simulink model "modelsimulator"  (R2023b)
settings: Solver=VariableStepAuto  StartTime=0.0  StopTime=185  FixedStep=0.0002  RelTol=1e-3
values from neighbouring files (symbols this model uses):
  eta_init = [0 0 0 0 0 0]    [Linearization_validation.m]    (also in ROV_simulation_init.m = [radius 0 0 0 0 -pi/2])
  K_full = lqr(linsysROV_lqr,Q,R)    [ROV_simulation_init.m]
  K_reduced = lqr(linsysROV_lqr_reduced_disc,Q,R)    [ROV_simulation_init.m]
  omega = 0.0174532925*5    (= 0.0872664625)    [ROV_simulation_init.m]
  p = [-125.691529893755	-8.50647884753240	275.922008410927	13.4112646958028	-226.567986780204	-3.28875901062827	118.657519470084	6.62648580653865	14.9826070833980	0.00]    [ROV_simulation_init.m]
  PID_phi = [11.6676, 5.8503, -12.3688, 0.025226,34]    [ROV_simulation_init.m]
  PID_psi = [11.3054, 1.000, -3.8005, 0.087502,30]    [ROV_simulation_init.m]
  PID_theta = [10.2974, 5.9702, -15.653, 0.016423,19]    [ROV_simulation_init.m]
  PID_x = [500.411, 30.5093, -500.8638, 0.032394,110]    [ROV_simulation_init.m]
  PID_y = [500.7275, 20.1075, -500.8002, 0.019369,110]    [ROV_simulation_init.m]
  PID_z = [500.7655, 25.0859, -500.5557, 0.026709,158]    [ROV_simulation_init.m]
  radius = 5    [ROV_simulation_init.m]
  ROV = initializeModelMatrices(m,I,COG,l,w,h,Thrusters)    [CreateGramianROV.m]    (also in CreateROVLin.m = initializeModelMatrices(m, I, COB, dim, BlueROVHeavy); Eigenvalue_tracking.m = initializeModelMatrices(m, I, COB,dim,0); Linearization_validation.m = initializeModelMatrices(m, I, COB,dim,0); ROV_simulation_init.m = initializeModelMatrices(m, Inertia, COB, dim, BlueROVHeavy))
  T_inv = ROV.T'/(ROV.T*ROV.T')    [ROV_simulation_init.m]
  ThrusterVoltage = 14    [ROV_simulation_init.m]
  v_init = [3 0 0 0 0 0]    [Linearization_validation.m]    (also in ROV_simulation_init.m = [omega omega z_rate 0 0 omega])
  z_rate = 0.1    [ROV_simulation_init.m]
libraries: simulink x60
(part 3 of 3)

== matlab function modelsimulator/PID/Tau_body/InvNED ==
  data: Tau1 input; x_dot output; Tau2 input; Tau3 input; Tau4 input; Tau5 input; Tau6 input; x input; y input; z input; phi input; theta input; pzi input; y_dot output; z_dot output; phi_dot output; theta_dot output; pzi_dot output
function [x_dot,y_dot,z_dot,phi_dot,theta_dot,pzi_dot] = InvNED(Tau1,Tau2,Tau3,Tau4,Tau5,Tau6,x,y,z,phi,theta,pzi)
%#codegen

%    This function was generated by the Symbolic Math Toolbox version 23.2.
%    07-Jun-2024 11:07:48

% Tau1 = complex(Tau1);  % if required to enforce complex operations
% Tau2 = complex(Tau2);  % if required to enforce complex operations
% Tau3 = complex(Tau3);  % if required to enforce complex operations
% Tau4 = complex(Tau4);  % if required to enforce complex operations
% Tau5 = complex(Tau5);  % if required to enforce complex operations
% Tau6 = complex(Tau6);  % if required to enforce complex operations
% x = complex(x);  % if required to enforce complex operations
% y = complex(y);  % if required to enforce complex operations
% z = complex(z);  % if required to enforce complex operations
% phi = complex(phi);  % if required to enforce complex operations
% theta = complex(theta);  % if required to enforce complex operations
% pzi = complex(pzi);  % if required to enforce complex operations
t2 = cos(phi);
t3 = cos(pzi);
t4 = cos(theta);
t5 = sin(phi);
t6 = sin(pzi);
t7 = sin(theta);
t8 = t2.^2;
t9 = t3.^2;
t10 = t4.^2;
t11 = t5.^2;
t12 = t6.^2;
t13 = t7.^2;
t14 = t8.*t10;
t15 = t8+t11;
t16 = t9+t12;
t17 = t8.*t13;
t18 = t10.*t11;
t19 = t11.*t13;
t20 = 1.0./t15;
t21 = 1.0./t16;
x_dot = (t21.*(Tau1.*t3.*t4+Tau2.*t4.*t6-Tau3.*t7.*t9-Tau3.*t7.*t12))./(t10+t13);
if nargout > 1
    t22 = t14+t17+t18+t19;
    t23 = 1.0./t22;
    y_dot = t21.*t23.*(Tau1.*t3.*t5.*t7+Tau2.*t2.*t3.*t10-Tau1.*t2.*t6.*t10+Tau2.*t2.*t3.*t13+Tau2.*t5.*t6.*t7+Tau3.*t4.*t5.*t9-Tau1.*t2.*t6.*t13+Tau3.*t4.*t5.*t12);
end
if nargout > 2
    z_dot = t21.*t23.*(Tau1.*t2.*t3.*t7+Tau2.*t2.*t6.*t7+Tau3.*t2.*t4.*t9-Tau2.*t3.*t5.*t10+Tau3.*t2.*t4.*t12+Tau1.*t5.*t6.*t10-Tau2.*t3.*t5.*t13+Tau1.*t5.*t6.*t13);
end
if nargout > 3
    phi_dot = Tau4-Tau6.*t4.*tan(theta);
end
if nargout > 4
    theta_dot = t20.*(Tau5.*t2+Tau6.*t4.*t5);
end
if nargout > 5
    pzi_dot = -t20.*(Tau5.*t5-Tau6.*t2.*t4);
end
end

== matlab function modelsimulator/LQR_full/Tau_body/InvNED ==
  data: Tau1 input; x_dot output; Tau2 input; Tau3 input; Tau4 input; Tau5 input; Tau6 input; x input; y input; z input; phi input; theta input; pzi input; y_dot output; z_dot output; phi_dot output; theta_dot output; pzi_dot output
function [x_dot,y_dot,z_dot,phi_dot,theta_dot,pzi_dot] = InvNED(Tau1,Tau2,Tau3,Tau4,Tau5,Tau6,x,y,z,phi,theta,pzi)
%#codegen

%    This function was generated by the Symbolic Math Toolbox version 23.2.
%    21-May-2024 16:03:04

% Tau1 = complex(Tau1);  % if required to enforce complex operations
% Tau2 = complex(Tau2);  % if required to enforce complex operations
% Tau3 = complex(Tau3);  % if required to enforce complex operations
% Tau4 = complex(Tau4);  % if required to enforce complex operations
% Tau5 = complex(Tau5);  % if required to enforce complex operations
% Tau6 = complex(Tau6);  % if required to enforce complex operations
% x = complex(x);  % if required to enforce complex operations
% y = complex(y);  % if required to enforce complex operations
% z = complex(z);  % if required to enforce complex operations
% phi = complex(phi);  % if required to enforce complex operations
% theta = complex(theta);  % if required to enforce complex operations
% pzi = complex(pzi);  % if required to enforce complex operations
t2 = cos(phi);
t3 = cos(pzi);
t4 = cos(theta);
t5 = sin(phi);
t6 = sin(pzi);
t7 = sin(theta);
t8 = t2.^2;
t9 = t3.^2;
t10 = t4.^2;
t11 = t5.^2;
t12 = t6.^2;
t13 = t7.^2;
t14 = t8.*t10;
t15 = t8+t11;
t16 = t9+t12;
t17 = t8.*t13;
t18 = t10.*t11;
t19 = t11.*t13;
t20 = 1.0./t15;
t21 = 1.0./t16;
x_dot = (t21.*(Tau1.*t3.*t4+Tau2.*t4.*t6-Tau3.*t7.*t9-Tau3.*t7.*t12))./(t10+t13);
if nargout > 1
    t22 = t14+t17+t18+t19;
    t23 = 1.0./t22;
    y_dot = t21.*t23.*(Tau1.*t3.*t5.*t7+Tau2.*t2.*t3.*t10-Tau1.*t2.*t6.*t10+Tau2.*t2.*t3.*t13+Tau2.*t5.*t6.*t7+Tau3.*t4.*t5.*t9-Tau1.*t2.*t6.*t13+Tau3.*t4.*t5.*t12);
end
if nargout > 2
    z_dot = t21.*t23.*(Tau1.*t2.*t3.*t7+Tau2.*t2.*t6.*t7+Tau3.*t2.*t4.*t9-Tau2.*t3.*t5.*t10+Tau3.*t2.*t4.*t12+Tau1.*t5.*t6.*t10-Tau2.*t3.*t5.*t13+Tau1.*t5.*t6.*t13);
end
if nargout > 3
    phi_dot = Tau4-Tau6.*t4.*tan(theta);
end
if nargout > 4
    theta_dot = t20.*(Tau5.*t2+Tau6.*t4.*t5);
end
if nargout > 5
    pzi_dot = -t20.*(Tau5.*t5-Tau6.*t2.*t4);
end
end

== matlab function modelsimulator/SMC/SMC_internal/SMC ==
  data: x input; Tau_1 output; y input; z input; phi input; theta input; pzi input; x_d input; y_d input; z_d input; phi_d input; theta_d input; pzi_d input; ref1 input; ref2 input; ref3 input; ref4 input; ref5 input; ref6 input; ref_d1 input; ref_d2 input; ref_d3 input; ref_d4 input; ref_d5 input; ref_d6 input; ref_dd1 input; ref_dd2 input; ref_dd3 input; ref_dd4 input; ref_dd5 input; ref_dd6 input; Tau_2 output; Tau_3 output; Tau_4 output; Tau_5 output; Tau_6 output; e_int1 input; e_int2 input; e_int3 input; e_int4 input; e_int5 input; e_int6 input; S_1 output; S_2 output; S_3 output; S_4 output; S_5 output; S_6 output
function [Tau_1,Tau_2,Tau_3,Tau_4,Tau_5,Tau_6,S_1,S_2,S_3,S_4,S_5,S_6] = SMC(x,y,z,phi,theta,pzi,x_d,y_d,z_d,phi_d,theta_d,pzi_d,ref1,ref2,ref3,ref4,ref5,ref6,ref_d1,ref_d2,ref_d3,ref_d4,ref_d5,ref_d6,ref_dd1,ref_dd2,ref_dd3,ref_dd4,ref_dd5,ref_dd6,e_int1,e_int2,e_int3,e_int4,e_int5,e_int6)
%#codegen

%    This function was generated by the Symbolic Math Toolbox version 23.2.
%    07-Jun-2024 11:09:30

% x = complex(x);  % if required to enforce complex operations
% y = complex(y);  % if required to enforce complex operations
% z = complex(z);  % if required to enforce complex operations
% phi = complex(phi);  % if required to enforce complex operations
% theta = complex(theta);  % if required to enforce complex operations
% pzi = complex(pzi);  % if required to enforce complex operations
% x_d = complex(x_d);  % if required to enforce complex operations
% y_d = complex(y_d);  % if required to enforce complex operations
% z_d = complex(z_d);  % if required to enforce complex operations
% phi_d = complex(phi_d);  % if required to enforce complex operations
% theta_d = complex(theta_d);  % if required to enforce complex operations
% pzi_d = complex(pzi_d);  % if required to enforce complex operations
% ref1 = complex(ref1);  % if required to enforce complex operations
% ref2 = complex(ref2);  % if required to enforce complex operations
% ref3 = complex(ref3);  % if required to enforce complex operations
% ref4 = complex(ref4);  % if required to enforce complex operations
% ref5 = complex(ref5);  % if required to enforce complex operations
% ref6 = complex(ref6);  % if required to enforce complex operations
% ref_d1 = complex(ref_d1);  % if required to enforce complex operations
% ref_d2 = complex(ref_d2);  % if required to enforce complex operations
% ref_d3 = complex(ref_d3);  % if required to enforce complex operations
% ref_d4 = complex(ref_d4);  % if required to enforce complex operations
% ref_d5 = complex(ref_d5);  % if required to enforce complex operations
% ref_d6 = complex(ref_d6);  % if required to enforce complex operations
% ref_dd1 = complex(ref_dd1);  % if required to enforce complex operations
% ref_dd2 = complex(ref_dd2);  % if required to enforce complex operations
% ref_dd3 = complex(ref_dd3);  % if required to enforce complex operations
% ref_dd4 = complex(ref_dd4);  % if required to enforce complex operations
% ref_dd5 = complex(ref_dd5);  % if required to enforce complex operations
% ref_dd6 = complex(ref_dd6);  % if required to enforce complex operations
% e_int1 = complex(e_int1);  % if required to enforce complex operations
% e_int2 = complex(e_int2);  % if required to enforce complex operations
% e_int3 = complex(e_int3);  % if required to enforce complex operations
% e_int4 = complex(e_int4);  % if required to enforce complex operations
% e_int5 = complex(e_int5);  % if required to enforce complex operations
% e_int6 = complex(e_int6);  % if required to enforce complex operations
t2 = abs(phi_d);
t3 = abs(pzi_d);
t4 = cos(phi);
t5 = cos(pzi);
t6 = abs(theta_d);
t7 = cos(theta);
t8 = abs(x_d);
t9 = abs(y_d);
t10 = abs(z_d);
t11 = sin(phi);
t12 = sin(pzi);
t13 = sin(theta);
t14 = tan(theta);
t15 = ref1.*2.0;
t16 = ref2.*2.0;
t17 = ref3.*2.0;
t18 = x.*2.0;
t19 = y.*2.0;
t20 = z.*2.0;
t35 = -ref_d1;
t36 = -ref_d2;
t37 = -ref_d3;
t38 = -ref_d4;
t39 = -ref_d5;
t40 = -ref_d6;
t41 = e_int6./2.0;
t42 = ref5.*(7.0./2.0);
t43 = theta.*(7.0./2.0);
t44 = e_int1.*(3.0./2.0e+1);
t45 = e_int2.*(3.0./2.0e+1);
t46 = e_int3.*(3.0./2.0e+1);
t48 = e_int4.*(9.0./1.0e+1);
t49 = e_int5.*(2.1e+1./2.0e+1);
t50 = phi.*(2.7e+1./1.0e+1);
t51 = pzi.*(1.3e+1./1.0e+1);
t52 = ref6.*(1.3e+1./1.0e+1);
t53 = ref4.*(2.7e+1./1.0e+1);
t21 = t4.^2;
t22 = t5.^2;
t23 = t5.^3;
t24 = t7.^2;
t25 = t7.^3;
t26 = t11.^2;
t27 = t11.^3;
t28 = t12.^2;
t29 = t12.^3;
t30 = t13.^2;
t31 = t13.^3;
t32 = -t15;
t33 = -t16;
t34 = -t17;
t47 = -t42;
t54 = -t52;
t55 = -t53;
t56 = t21+t26;
t58 = t21.*t22.*t30;
t59 = t21.*t24.*t28;
t60 = t22.*t24.*t26;
t61 = t4.*t5.*t11.*t12.*t31;
t62 = t5.*t7.*t11.*t12.*t31;
t63 = t5.*t11.*t12.*t13.*t25;
t64 = t22.*t26.*t30;
t65 = t24.*t26.*t28;
t66 = t26.*t28.*t30;
t67 = t4.*t7.*t28.*t30;
t68 = t21.*t22.*t24;
t71 = t4.*t5.*t11.*t12.*t13.*t24;
t72 = t18+t32+t35+t44+x_d;
t73 = t19+t33+t36+t45+y_d;
t74 = t20+t34+t37+t46+z_d;
t75 = t39+t43+t47+t49+theta_d;
t76 = pzi_d+t40+t41+t51+t54;
t77 = phi_d+t38+t48+t50+t55;
t57 = 1.0./t56;
t69 = -t62;
t70 = -t63;
t78 = t58+t59+t60+t61+t64+t65+t66+t67+t68+t69+t70+t71;
t79 = 1.0./t78;
et1 = t58.*x_d.*4.50486366e+9+t60.*x_d.*3.031307621e+9+t61.*x_d.*4.50486366e+9-t63.*x_d.*3.031307621e+9+t65.*x_d.*4.50486366e+9+t66.*x_d.*4.50486366e+9+t68.*x_d.*3.031307621e+9+t71.*x_d.*7.536171281e+9+t8.*t60.*x_d.*3.119812953e+10+t9.*t59.*x_d.*4.62422226e+10+t10.*t58.*x_d.*2.59370938e+10-t8.*t63.*x_d.*3.119812953e+10-t9.*t62.*x_d.*4.62422226e+10+t10.*t61.*x_d.*2.59370938e+10;
et2 = t9.*t64.*x_d.*4.62422226e+10+t10.*t65.*x_d.*2.59370938e+10+t8.*t68.*x_d.*3.119812953e+10+t9.*t67.*x_d.*4.62422226e+10+t10.*t66.*x_d.*2.59370938e+10+t8.*t71.*x_d.*3.119812953e+10-t9.*t71.*x_d.*4.62422226e+10+t10.*t71.*x_d.*2.59370938e+10+t4.*t11.*t13.*t28.*y_d.*4.50486366e+9+t5.*t12.*t21.*t24.*y_d.*3.031307621e+9-t5.*t12.*t24.*t26.*y_d.*1.473556039e+9-t4.*t11.*t22.*t31.*y_d.*4.50486366e+9;
et3 = t5.*t12.*t21.*t30.*y_d.*4.50486366e+9-t5.*t12.*t26.*t30.*y_d.*4.50486366e+9+t4.*t7.*t11.*t29.*z_d.*4.50486366e+9+t7.*t13.*t21.*t23.*z_d.*1.473556039e+9-t7.*t13.*t23.*t26.*z_d.*3.031307621e+9+t4.*t5.*t11.*t12.*t13.*x_d.*4.50486366e+9-t4.*t9.*t11.*t13.*t28.*y_d.*4.62422226e+10+t4.*t10.*t11.*t13.*t28.*y_d.*2.59370938e+10+t5.*t8.*t12.*t21.*t24.*y_d.*3.119812953e+10-t5.*t9.*t12.*t21.*t24.*y_d.*4.62422226e+10-t4.*t11.*t13.*t22.*t24.*y_d.*4.50486366e+9;
et4 = t5.*t8.*t12.*t24.*t26.*y_d.*3.119812953e+10+t4.*t9.*t11.*t22.*t31.*y_d.*4.62422226e+10-t5.*t9.*t12.*t21.*t30.*y_d.*4.62422226e+10-t5.*t10.*t12.*t24.*t26.*y_d.*2.59370938e+10-t4.*t10.*t11.*t22.*t31.*y_d.*2.59370938e+10+t5.*t10.*t12.*t21.*t30.*y_d.*2.59370938e+10+t5.*t9.*t12.*t26.*t30.*y_d.*4.62422226e+10-t5.*t10.*t12.*t26.*t30.*y_d.*2.59370938e+10+t4.*t7.*t11.*t12.*t22.*z_d.*4.50486366e+9-t4.*t7.*t9.*t11.*t29.*z_d.*4.62422226e+10;
et5 = t4.*t7.*t10.*t11.*t29.*z_d.*2.59370938e+10-t7.*t8.*t13.*t21.*t23.*z_d.*3.119812953e+10-t4.*t5.*t13.*t24.*t28.*z_d.*3.031307621e+9+t5.*t7.*t13.*t21.*t28.*z_d.*4.50486366e+9+t7.*t10.*t13.*t21.*t23.*z_d.*2.59370938e+10-t7.*t8.*t13.*t23.*t26.*z_d.*3.119812953e+10+t7.*t9.*t13.*t23.*t26.*z_d.*4.62422226e+10-t5.*t7.*t13.*t26.*t28.*z_d.*3.031307621e+9+t11.*t12.*t22.*t24.*t30.*z_d.*3.031307621e+9-t4.*t5.*t9.*t11.*t12.*t13.*x_d.*4.62422226e+10;
et6 = t4.*t5.*t10.*t11.*t12.*t13.*x_d.*2.59370938e+10+t4.*t9.*t11.*t13.*t22.*t24.*y_d.*4.62422226e+10-t4.*t10.*t11.*t13.*t22.*t24.*y_d.*2.59370938e+10-t4.*t7.*t9.*t11.*t12.*t22.*z_d.*4.62422226e+10+t4.*t7.*t10.*t11.*t12.*t22.*z_d.*2.59370938e+10-t4.*t5.*t8.*t13.*t24.*t28.*z_d.*3.119812953e+10+t4.*t5.*t9.*t13.*t24.*t28.*z_d.*4.62422226e+10-t5.*t7.*t9.*t13.*t21.*t28.*z_d.*4.62422226e+10+t5.*t7.*t10.*t13.*t21.*t28.*z_d.*2.59370938e+10-t4.*t7.*t11.*t12.*t22.*t30.*z_d.*3.031307621e+9;
et7 = t5.*t7.*t8.*t13.*t26.*t28.*z_d.*-3.119812953e+10+t5.*t7.*t9.*t13.*t26.*t28.*z_d.*4.62422226e+10+t8.*t11.*t12.*t22.*t24.*t30.*z_d.*3.119812953e+10-t9.*t11.*t12.*t22.*t24.*t30.*z_d.*4.62422226e+10-t4.*t7.*t8.*t11.*t12.*t22.*t30.*z_d.*3.119812953e+10+t4.*t7.*t9.*t11.*t12.*t22.*t30.*z_d.*4.62422226e+10;
Tau_1 = -(t72.*(abs(ref1.*(-3.0./2.0e+1)-ref_d1.*2.0+ref_dd1+x.*(3.0./2.0e+1)+x_d.*2.0+t79.*(et1+et2+et3+et4+et5+et6+et7).*2.275680623214713e-10).*(9.93e+2./5.0e+1)+9.93e+2./2.5e+1))./(abs(t72)+1.0./1.0e+1);
if nargout > 1
    et8 = t59.*y_d.*3.031307621e+9+t60.*y_d.*4.50486366e+9-t62.*y_d.*4.50486366e+9-t63.*y_d.*4.50486366e+9+t64.*y_d.*4.50486366e+9+t65.*y_d.*3.031307621e+9+t67.*y_d.*4.50486366e+9+t8.*t59.*y_d.*3.119812953e+10+t9.*t58.*y_d.*4.62422226e+10+t9.*t61.*y_d.*4.62422226e+10+t10.*t60.*y_d.*2.59370938e+10-t10.*t62.*y_d.*2.59370938e+10+t8.*t65.*y_d.*3.119812953e+10-t10.*t63.*y_d.*2.59370938e+10;
    et9 = t10.*t64.*y_d.*2.59370938e+10+t9.*t66.*y_d.*4.62422226e+10+t9.*t68.*y_d.*4.62422226e+10+t10.*t67.*y_d.*2.59370938e+10+t9.*t71.*y_d.*4.62422226e+10-t5.*t11.*t67.*z_d.*3.031307621e+9-t4.*t11.*t13.*t22.*x_d.*4.50486366e+9+t5.*t12.*t21.*t24.*x_d.*3.031307621e+9-t5.*t12.*t24.*t26.*x_d.*1.473556039e+9-t5.*t12.*t26.*t30.*x_d.*4.50486366e+9+t7.*t11.*t28.*t31.*x_d.*4.50486366e+9+t11.*t13.*t25.*t28.*x_d.*1.473556039e+9;
    et10 = t4.*t7.*t11.*t23.*z_d.*-4.50486366e+9+t4.*t13.*t24.*t29.*z_d.*1.473556039e+9-t7.*t13.*t26.*t29.*z_d.*3.031307621e+9-t5.*t8.*t11.*t67.*z_d.*3.119812953e+10+t5.*t9.*t11.*t67.*z_d.*4.62422226e+10+t4.*t5.*t7.*t12.*t30.*x_d.*4.50486366e+9+t4.*t9.*t11.*t13.*t22.*x_d.*4.62422226e+10-t4.*t10.*t11.*t13.*t22.*x_d.*2.59370938e+10+t5.*t8.*t12.*t21.*t24.*x_d.*3.119812953e+10-t5.*t9.*t12.*t21.*t24.*x_d.*4.62422226e+10+t5.*t8.*t12.*t24.*t26.*x_d.*3.119812953e+10;
    et11 = t5.*t10.*t12.*t24.*t26.*x_d.*-2.59370938e+10+t4.*t11.*t13.*t24.*t28.*x_d.*3.031307621e+9+t5.*t9.*t12.*t26.*t30.*x_d.*4.62422226e+10-t5.*t10.*t12.*t26.*t30.*x_d.*2.59370938e+10-t8.*t11.*t13.*t25.*t28.*x_d.*3.119812953e+10-t7.*t9.*t11.*t28.*t31.*x_d.*4.62422226e+10+t7.*t10.*t11.*t28.*t31.*x_d.*2.59370938e+10+t10.*t11.*t13.*t25.*t28.*x_d.*2.59370938e+10-t4.*t5.*t11.*t12.*t13.*y_d.*4.50486366e+9+t4.*t7.*t9.*t11.*t23.*z_d.*4.62422226e+10;
    et12 = t4.*t5.*t7.*t11.*t28.*z_d.*-4.50486366e+9-t4.*t7.*t10.*t11.*t23.*z_d.*2.59370938e+10+t4.*t12.*t13.*t22.*t24.*z_d.*4.50486366e+9-t7.*t12.*t13.*t21.*t22.*z_d.*3.031307621e+9-t4.*t8.*t13.*t24.*t29.*z_d.*3.119812953e+10+t4.*t10.*t13.*t24.*t29.*z_d.*2.59370938e+10-t7.*t12.*t13.*t22.*t26.*z_d.*3.031307621e+9-t7.*t8.*t13.*t26.*t29.*z_d.*3.119812953e+10+t7.*t9.*t13.*t26.*t29.*z_d.*4.62422226e+10+t5.*t11.*t24.*t28.*t30.*z_d.*3.031307621e+9;
    et13 = t4.*t5.*t7.*t9.*t12.*t30.*x_d.*-4.62422226e+10+t4.*t5.*t7.*t10.*t12.*t30.*x_d.*2.59370938e+10+t4.*t8.*t11.*t13.*t24.*t28.*x_d.*3.119812953e+10-t4.*t9.*t11.*t13.*t24.*t28.*x_d.*4.62422226e+10+t4.*t5.*t9.*t11.*t12.*t13.*y_d.*4.62422226e+10-t4.*t5.*t10.*t11.*t12.*t13.*y_d.*2.59370938e+10+t4.*t5.*t7.*t9.*t11.*t28.*z_d.*4.62422226e+10-t4.*t5.*t7.*t10.*t11.*t28.*z_d.*2.59370938e+10-t7.*t8.*t12.*t13.*t21.*t22.*z_d.*3.119812953e+10-t4.*t9.*t12.*t13.*t22.*t24.*z_d.*4.62422226e+10;
    et14 = t7.*t9.*t12.*t13.*t21.*t22.*z_d.*4.62422226e+10+t4.*t10.*t12.*t13.*t22.*t24.*z_d.*2.59370938e+10-t7.*t8.*t12.*t13.*t22.*t26.*z_d.*3.119812953e+10+t7.*t9.*t12.*t13.*t22.*t26.*z_d.*4.62422226e+10+t5.*t8.*t11.*t24.*t28.*t30.*z_d.*3.119812953e+10-t5.*t9.*t11.*t24.*t28.*t30.*z_d.*4.62422226e+10;
    Tau_2 = -(t73.*(abs(ref2.*(-3.0./2.0e+1)-ref_d2.*2.0+ref_dd2+y.*(3.0./2.0e+1)+y_d.*2.0+t79.*(et8+et9+et10+et11+et12+et13+et14).*2.275680623214713e-10).*2.0621e+1+4.124e+1))./(abs(t73)+1.0./1.0e+1);
end
if nargout > 2
    et15 = t58.*z_d.*3.031307621e+9+t59.*z_d.*4.50486366e+9+t61.*z_d.*3.031307621e+9-t62.*z_d.*3.031307621e+9+t64.*z_d.*3.031307621e+9+t66.*z_d.*3.031307621e+9+t67.*z_d.*3.031307621e+9+t68.*z_d.*4.50486366e+9+t8.*t58.*z_d.*3.119812953e+10+t8.*t61.*z_d.*3.119812953e+10+t9.*t60.*z_d.*4.62422226e+10+t10.*t59.*z_d.*2.59370938e+10-t8.*t62.*z_d.*3.119812953e+10+t8.*t64.*z_d.*3.119812953e+10;
    et16 = t9.*t63.*z_d.*-4.62422226e+10+t8.*t66.*z_d.*3.119812953e+10+t9.*t65.*z_d.*4.62422226e+10+t8.*t67.*z_d.*3.119812953e+10+t10.*t68.*z_d.*2.59370938e+10+t9.*t71.*z_d.*4.62422226e+10+t5.*t7.*t13.*t21.*x_d.*1.473556039e+9-t5.*t7.*t13.*t26.*x_d.*3.031307621e+9+t4.*t11.*t12.*t25.*x_d.*4.50486366e+9+t11.*t12.*t24.*t30.*x_d.*3.031307621e+9-t4.*t5.*t11.*t25.*y_d.*4.50486366e+9+t7.*t12.*t13.*t21.*y_d.*1.473556039e+9;
    et17 = t7.*t12.*t13.*t26.*y_d.*-3.031307621e+9-t5.*t7.*t8.*t13.*t21.*x_d.*3.119812953e+10+t5.*t7.*t10.*t13.*t21.*x_d.*2.59370938e+10-t5.*t7.*t8.*t13.*t26.*x_d.*3.119812953e+10+t5.*t7.*t9.*t13.*t26.*x_d.*4.62422226e+10-t4.*t9.*t11.*t12.*t25.*x_d.*4.62422226e+10+t4.*t10.*t11.*t12.*t25.*x_d.*2.59370938e+10+t4.*t7.*t11.*t12.*t30.*x_d.*1.473556039e+9+t8.*t11.*t12.*t24.*t30.*x_d.*3.119812953e+10-t9.*t11.*t12.*t24.*t30.*x_d.*4.62422226e+10+t4.*t5.*t9.*t11.*t25.*y_d.*4.62422226e+10;
    et18 = t4.*t5.*t10.*t11.*t25.*y_d.*-2.59370938e+10-t4.*t5.*t7.*t11.*t30.*y_d.*4.50486366e+9-t7.*t8.*t12.*t13.*t21.*y_d.*3.119812953e+10+t7.*t10.*t12.*t13.*t21.*y_d.*2.59370938e+10-t7.*t8.*t12.*t13.*t26.*y_d.*3.119812953e+10+t7.*t9.*t12.*t13.*t26.*y_d.*4.62422226e+10-t4.*t7.*t8.*t11.*t12.*t30.*x_d.*3.119812953e+10+t4.*t7.*t10.*t11.*t12.*t30.*x_d.*2.59370938e+10+t4.*t5.*t7.*t9.*t11.*t30.*y_d.*4.62422226e+10-t4.*t5.*t7.*t10.*t11.*t30.*y_d.*2.59370938e+10;
    Tau_3 = -(t74.*(abs(ref3.*(-3.0./2.0e+1)-ref_d3.*2.0+ref_dd3+z.*(3.0./2.0e+1)+z_d.*2.0+t79.*(et15+et16+et17+et18).*2.275680623214713e-10).*3.219e+1+4.828e+1))./(abs(t74)+1.0./1.0e+1);
end
if nargout > 3
    et19 = t7.*t27.*9.535282848e+9+phi_d.*t2.*t21.*8.57362688e+9+phi_d.*t2.*t26.*8.57362688e+9+t7.*t11.*t21.*9.535282848e+9+t13.*t14.*t27.*1.1652492033e+10+pzi_d.*t7.*t14.*t26.*7.031752e+9+t11.*t13.*t14.*t21.*1.1652492033e+10+t4.*t11.*t14.*theta_d.*7.031752e+9-pzi_d.*t2.*t7.*t14.*t21.*8.57362688e+9+pzi_d.*t3.*t7.*t14.*t21.*8.131392e+9-pzi_d.*t2.*t7.*t14.*t26.*8.57362688e+9+pzi_d.*t6.*t7.*t14.*t26.*4.1311543e+9;
    et20 = t3.*t4.*t11.*t14.*theta_d.*-8.131392e+9+t4.*t6.*t11.*t14.*theta_d.*4.1311543e+9;
    Tau_4 = -(t77.*(abs(phi.*(9.0./1.0e+1)+phi_d.*(2.7e+1./1.0e+1)-ref4.*(9.0./1.0e+1)-ref_d4.*(2.7e+1./1.0e+1)+ref_dd4+(t57.*(et19+et20))./3.206478912e+9).*4.458e-1+6.3e+1./2.0e+1))./(abs(t77)+3.0./1.0e+1);
end
if nargout > 4
    Tau_5 = -(t75.*(abs(ref5.*(-2.1e+1./2.0e+1)-ref_d5.*(7.0./2.0)+ref_dd5+theta.*(2.1e+1./2.0e+1)+theta_d.*(7.0./2.0)+(t57.*(t21.*theta_d.*9.464e+6+t4.^3.*t13.*1.5683031e+7+t4.*t13.*t26.*1.5683031e+7+t6.*t21.*theta_d.*5.5601e+6+t3.*t26.*theta_d.*1.0944e+7+pzi_d.*t4.*t7.*t11.*9.464e+6-pzi_d.*t3.*t4.*t7.*t11.*1.0944e+7+pzi_d.*t4.*t6.*t7.*t11.*5.5601e+6))./4.315584e+6).*(2.28e+2./6.25e+2)+7.2e+1./2.5e+1))./(abs(t75)+3.0./1.0e+1);
end
if nargout > 5
    Tau_6 = -(t76.*(abs(pzi./2.0+pzi_d.*(1.3e+1./1.0e+1)-ref6./2.0-ref_d6.*(1.3e+1./1.0e+1)+ref_dd6+(t57.*(t13.*t27.*1.5683031e+7+pzi_d.*t7.*t26.*9.464e+6+t11.*t13.*t21.*1.5683031e+7+t4.*t11.*theta_d.*9.464e+6+pzi_d.*t3.*t7.*t21.*1.0944e+7+pzi_d.*t6.*t7.*t26.*5.5601e+6-t3.*t4.*t11.*theta_d.*1.0944e+7+t4.*t6.*t11.*theta_d.*5.5601e+6))./(t7.*4.315584e+6)).*5.915e-1+3.9e+1./2.0e+1))./(abs(t76)+1.0./5.0);
end
if nargout > 6
    S_1 = t72;
end
if nargout > 7
    S_2 = t73;
end
if nargout > 8
    S_3 = t74;
end
if nargout > 9
    S_4 = t77;
end
if nargout > 10
    S_5 = t75;
end
if nargout > 11
    S_6 = t76;
end
end

== matlab function modelsimulator/SMC/Tau_body/InvNED ==
  data: u input; x_dot output; v input; w input; p input; q input; r input; x input; y input; z input; phi input; theta input; pzi input; y_dot output; z_dot output; phi_dot output; theta_dot output; pzi_dot output
function [x_dot,y_dot,z_dot,phi_dot,theta_dot,pzi_dot] = InvNED(u,v,w,p,q,r,x,y,z,phi,theta,pzi)
%#codegen

%    This function was generated by the Symbolic Math Toolbox version 23.2.
%    09-May-2024 13:14:03

% u = complex(u);  % if required to enforce complex operations
% v = complex(v);  % if required to enforce complex operations
% w = complex(w);  % if required to enforce complex operations
% p = complex(p);  % if required to enforce complex operations
% q = complex(q);  % if required to enforce complex operations
% r = complex(r);  % if required to enforce complex operations
% x = complex(x);  % if required to enforce complex operations
% y = complex(y);  % if required to enforce complex operations
% z = complex(z);  % if required to enforce complex operations
% phi = complex(phi);  % if required to enforce complex operations
% theta = complex(theta);  % if required to enforce complex operations
% pzi = complex(pzi);  % if required to enforce complex operations
t2 = cos(phi);
t3 = cos(pzi);
t4 = cos(theta);
t5 = sin(phi);
t6 = sin(pzi);
t7 = sin(theta);
t8 = t2.^2;
t9 = t3.^2;
t10 = t4.^2;
t11 = t5.^2;
t12 = t6.^2;
t13 = t7.^2;
t14 = t8.*t10;
t15 = t8+t11;
t16 = t9+t12;
t17 = t8.*t13;
t18 = t10.*t11;
t19 = t11.*t13;
t20 = 1.0./t15;
t21 = 1.0./t16;
x_dot = (t21.*(t3.*t4.*u+t4.*t6.*v-t7.*t9.*w-t7.*t12.*w))./(t10+t13);
if nargout > 1
    t22 = t14+t17+t18+t19;
    t23 = 1.0./t22;
    y_dot = t21.*t23.*(t3.*t5.*t7.*u-t2.*t6.*t10.*u-t2.*t6.*t13.*u+t2.*t3.*t10.*v+t2.*t3.*t13.*v+t5.*t6.*t7.*v+t4.*t5.*t9.*w+t4.*t5.*t12.*w);
end
if nargout > 2
    z_dot = t21.*t23.*(t2.*t3.*t7.*u+t5.*t6.*t10.*u+t5.*t6.*t13.*u+t2.*t6.*t7.*v-t3.*t5.*t10.*v-t3.*t5.*t13.*v+t2.*t4.*t9.*w+t2.*t4.*t12.*w);
end
if nargout > 3
    phi_dot = p-r.*t4.*tan(theta);
end
if nargout > 4
    theta_dot = t20.*(q.*t2+r.*t4.*t5);
end
if nargout > 5
    pzi_dot = -t20.*(q.*t5-r.*t2.*t4);
end
end

== matlab function modelsimulator/ROV1/NED/calcNED ==
  data: u input; x_dot output; v input; w input; p input; q input; r input; x input; y input; z input; phi input; theta input; pzi input; y_dot output; z_dot output; phi_dot output; theta_dot output; pzi_dot output
function [x_dot,y_dot,z_dot,phi_dot,theta_dot,pzi_dot] = calcNED(u,v,w,p,q,r,x,y,z,phi,theta,pzi)
%#codegen

%    This function was generated by the Symbolic Math Toolbox version 23.2.
%    12-May-2024 11:32:59

% u = complex(u);  % if required to enforce complex operations
% v = complex(v);  % if required to enforce complex operations
% w = complex(w);  % if required to enforce complex operations
% p = complex(p);  % if required to enforce complex operations
% q = complex(q);  % if required to enforce complex operations
% r = complex(r);  % if required to enforce complex operations
% x = complex(x);  % if required to enforce complex operations
% y = complex(y);  % if required to enforce complex operations
% z = complex(z);  % if required to enforce complex operations
% phi = complex(phi);  % if required to enforce complex operations
% theta = complex(theta);  % if required to enforce complex operations
% pzi = complex(pzi);  % if required to enforce complex operations
t2 = cos(phi);
t3 = cos(pzi);
t4 = cos(theta);
t5 = sin(phi);
t6 = sin(pzi);
t7 = sin(theta);
x_dot = -v.*(t2.*t6-t3.*t5.*t7)+w.*(t5.*t6+t2.*t3.*t7)+t3.*t4.*u;
if nargout > 1
    y_dot = v.*(t2.*t3+t5.*t6.*t7)-w.*(t3.*t5-t2.*t6.*t7)+t4.*t6.*u;
end
if nargout > 2
    z_dot = -t7.*u+t4.*t5.*v+t2.*t4.*w;
end
if nargout > 3
    t8 = tan(theta);
    phi_dot = p+q.*t5.*t8+r.*t2.*t8;
end
if nargout > 4
    theta_dot = q.*t2-r.*t5;
end
if nargout > 5
    t9 = 1.0./t4;
    pzi_dot = q.*t5.*t9+r.*t2.*t9;
end
end

== matlab function modelsimulator/ROV1/NED1/calcNED ==
  data: u input; x_dot output; v input; w input; p input; q input; r input; x input; y input; z input; phi input; theta input; pzi input; y_dot output; z_dot output; phi_dot output; theta_dot output; pzi_dot output
function [x_dot,y_dot,z_dot,phi_dot,theta_dot,pzi_dot] = calcNED(u,v,w,p,q,r,x,y,z,phi,theta,pzi)
%#codegen

%    This function was generated by the Symbolic Math Toolbox version 23.2.
%    06-May-2024 15:56:40

% u = complex(u);  % if required to enforce complex operations
% v = complex(v);  % if required to enforce complex operations
% w = complex(w);  % if required to enforce complex operations
% p = complex(p);  % if required to enforce complex operations
% q = complex(q);  % if required to enforce complex operations
% r = complex(r);  % if required to enforce complex operations
% x = complex(x);  % if required to enforce complex operations
% y = complex(y);  % if required to enforce complex operations
% z = complex(z);  % if required to enforce complex operations
% phi = complex(phi);  % if required to enforce complex operations
% theta = complex(theta);  % if required to enforce complex operations
% pzi = complex(pzi);  % if required to enforce complex operations
t2 = cos(phi);
t3 = cos(pzi);
t4 = cos(theta);
t5 = sin(phi);
t6 = sin(pzi);
t7 = sin(theta);
x_dot = -v.*(t2.*t6-t3.*t5.*t7)+w.*(t5.*t6+t2.*t3.*t7)+t3.*t4.*u;
if nargout > 1
    y_dot = v.*(t2.*t3+t5.*t6.*t7)-w.*(t3.*t5-t2.*t6.*t7)+t4.*t6.*u;
end
if nargout > 2
    z_dot = -t7.*u+t4.*t5.*v+t2.*t4.*w;
end
if nargout > 3
    t8 = tan(theta);
    phi_dot = p+q.*t5.*t8+r.*t2.*t8;
end
if nargout > 4
    theta_dot = q.*t2-r.*t5;
end
if nargout > 5
    t9 = 1.0./t4;
    pzi_dot = q.*t5.*t9+r.*t2.*t9;
end
end

== matlab function modelsimulator/ROV1/ROVSubsystem/ROV ==
  data: u input; u_dot output; v input; w input; p input; q input; r input; x input; y input; z input; phi input; theta input; pzi input; tau1 input; tau2 input; tau3 input; tau4 input; tau5 input; tau6 input; v_dot output; w_dot output; p_dot output; q_dot output; r_dot output
function [u_dot,v_dot,w_dot,p_dot,q_dot,r_dot] = ROV(u,v,w,p,q,r,x,y,z,phi,theta,pzi,tau1,tau2,tau3,tau4,tau5,tau6)
%#codegen

%    This function was generated by the Symbolic Math Toolbox version 23.2.
%    07-Jun-2024 11:07:46

% u = complex(u);  % if required to enforce complex operations
% v = complex(v);  % if required to enforce complex operations
% w = complex(w);  % if required to enforce complex operations
% p = complex(p);  % if required to enforce complex operations
% q = complex(q);  % if required to enforce complex operations
% r = complex(r);  % if required to enforce complex operations
% x = complex(x);  % if required to enforce complex operations
% y = complex(y);  % if required to enforce complex operations
% z = complex(z);  % if required to enforce complex operations
% phi = complex(phi);  % if required to enforce complex operations
% theta = complex(theta);  % if required to enforce complex operations
% pzi = complex(pzi);  % if required to enforce complex operations
% tau1 = complex(tau1);  % if required to enforce complex operations
% tau2 = complex(tau2);  % if required to enforce complex operations
% tau3 = complex(tau3);  % if required to enforce complex operations
% tau4 = complex(tau4);  % if required to enforce complex operations
% tau5 = complex(tau5);  % if required to enforce complex operations
% tau6 = complex(tau6);  % if required to enforce complex operations
u_dot = tau1.*(5.0e+1./9.93e+2)-u.*(6.85e+2./9.93e+2)-q.*w.*1.620845921450151+r.*v.*1.038318227593152-u.*abs(u).*7.099697885196375;
if nargout > 1
    v_dot = tau2.*4.849425343096843e-2+p.*w.*1.561030017942874-r.*u.*9.63095873139033e-1-v.*abs(v).*1.052325299452015e+1;
end
if nargout > 2
    w_dot = tau3.*3.106554830692762e-2-w.*1.025163094128611-p.*v.*6.406026716371544e-1+q.*u.*6.169617893755825e-1-w.*abs(w).*5.902454178316247;
end
if nargout > 3
    p_dot = tau4.*2.243158366980709-cos(theta).*sin(phi).*2.973755047106326-q.*r.*5.085240017945267e-1-v.*w.*2.595109914759982e+1-p.*abs(p).*2.673844773441005;
end
if nargout > 4
    q_dot = q.*(-1.25e+2./5.7e+1)+tau5.*(6.25e+2./2.28e+2)-sin(theta).*3.634046052631579+p.*r.*3.993969298245614e-1+u.*w.*3.379934210526316e+1-q.*abs(q).*1.288377192982456;
end
if nargout > 5
    r_dot = tau6.*1.69061707523246+p.*q.*1.369399830938292e-1-u.*v.*1.286559594251902-r.*abs(r).*2.53592561284869;
end
end

== matlab function modelsimulator/Thrusters_model1/MATLAB Function9 ==
  data: u input; F output; Thruster_voltage input
function F = fcn(u,Thruster_voltage)
if Thruster_voltage == 10
    p = [-92.7173526709009	-4.21942992652299	225.484550494853	8.63193834440817	-201.940923421530	-6.79855430208119	89.8300206612197	5.42728991500474	5.00491978379944	-0.00];
elseif Thruster_voltage == 12
    p = [-102.848572308239	-7.53059973031176	248.621713648981	14.4941570056757	-222.949976245640	-9.82587357024907	101.816137648126	6.80722654001185	7.78963212289893	-0.00];
elseif Thruster_voltage == 14
    p = [-111.940783464042	-6.65861599537878	269.823430407384	13.8659958797022	-243.064927768226	-10.2880091499065	114.063389337106	8.09188399656116	10.6145211900378	-0.00];
elseif Thruster_voltage == 16
    p =  [-148.575215521583	-6.01951344606880	347.062027953365	14.7939725163702	-299.865931981745	-13.0166356354772	134.177990099770	10.1629233711657	12.7092879704266	-0.00];
elseif Thruster_voltage == 18
    p = [-162.288059231193	-9.51335388922301	365.972527557958	19.4413549873700	-302.179637889150	-11.4404685775311	136.049916333434	8.61090564659817	14.1180490642860	-0.00];
elseif Thruster_voltage == 20
    p = [-125.691529893755	-8.50647884753240	275.922008410927	13.4112646958028	-226.567986780204	-3.28875901062827	118.657519470084	6.62648580653865	14.9826070833980	0.00];
else
    p = [0];
end
F = polyval(p,u);

== matlab function modelsimulator/ROV2/NED/calcNED ==
  data: u input; x_dot output; v input; w input; p input; q input; r input; x input; y input; z input; phi input; theta input; pzi input; y_dot output; z_dot output; phi_dot output; theta_dot output; pzi_dot output
function [x_dot,y_dot,z_dot,phi_dot,theta_dot,pzi_dot] = calcNED(u,v,w,p,q,r,x,y,z,phi,theta,pzi)
%#codegen

%    This function was generated by the Symbolic Math Toolbox version 23.2.
%    12-May-2024 11:32:59

% u = complex(u);  % if required to enforce complex operations
% v = complex(v);  % if required to enforce complex operations
% w = complex(w);  % if required to enforce complex operations
% p = complex(p);  % if required to enforce complex operations
% q = complex(q);  % if required to enforce complex operations
% r = complex(r);  % if required to enforce complex operations
% x = complex(x);  % if required to enforce complex operations
% y = complex(y);  % if required to enforce complex operations
% z = complex(z);  % if required to enforce complex operations
% phi = complex(phi);  % if required to enforce complex operations
% theta = complex(theta);  % if required to enforce complex operations
% pzi = complex(pzi);  % if required to enforce complex operations
t2 = cos(phi);
t3 = cos(pzi);
t4 = cos(theta);
t5 = sin(phi);
t6 = sin(pzi);
t7 = sin(theta);
x_dot = -v.*(t2.*t6-t3.*t5.*t7)+w.*(t5.*t6+t2.*t3.*t7)+t3.*t4.*u;
if nargout > 1
    y_dot = v.*(t2.*t3+t5.*t6.*t7)-w.*(t3.*t5-t2.*t6.*t7)+t4.*t6.*u;
end
if nargout > 2
    z_dot = -t7.*u+t4.*t5.*v+t2.*t4.*w;
end
if nargout > 3
    t8 = tan(theta);
    phi_dot = p+q.*t5.*t8+r.*t2.*t8;
end
if nargout > 4
    theta_dot = q.*t2-r.*t5;
end
if nargout > 5
    t9 = 1.0./t4;
    pzi_dot = q.*t5.*t9+r.*t2.*t9;
end
end

== matlab function modelsimulator/ROV2/NED1/calcNED ==
  data: u input; x_dot output; v input; w input; p input; q input; r input; x input; y input; z input; phi input; theta input; pzi input; y_dot output; z_dot output; phi_dot output; theta_dot output; pzi_dot output
function [x_dot,y_dot,z_dot,phi_dot,theta_dot,pzi_dot] = calcNED(u,v,w,p,q,r,x,y,z,phi,theta,pzi)
%#codegen

%    This function was generated by the Symbolic Math Toolbox version 23.2.
%    06-May-2024 15:56:40

% u = complex(u);  % if required to enforce complex operations
% v = complex(v);  % if required to enforce complex operations
% w = complex(w);  % if required to enforce complex operations
% p = complex(p);  % if required to enforce complex operations
% q = complex(q);  % if required to enforce complex operations
% r = complex(r);  % if required to enforce complex operations
% x = complex(x);  % if required to enforce complex operations
% y = complex(y);  % if required to enforce complex operations
% z = complex(z);  % if required to enforce complex operations
% phi = complex(phi);  % if required to enforce complex operations
% theta = complex(theta);  % if required to enforce complex operations
% pzi = complex(pzi);  % if required to enforce complex operations
t2 = cos(phi);
t3 = cos(pzi);
t4 = cos(theta);
t5 = sin(phi);
t6 = sin(pzi);
t7 = sin(theta);
x_dot = -v.*(t2.*t6-t3.*t5.*t7)+w.*(t5.*t6+t2.*t3.*t7)+t3.*t4.*u;
if nargout > 1
    y_dot = v.*(t2.*t3+t5.*t6.*t7)-w.*(t3.*t5-t2.*t6.*t7)+t4.*t6.*u;
end
if nargout > 2
    z_dot = -t7.*u+t4.*t5.*v+t2.*t4.*w;
end
if nargout > 3
    t8 = tan(theta);
    phi_dot = p+q.*t5.*t8+r.*t2.*t8;
end
if nargout > 4
    theta_dot = q.*t2-r.*t5;
end
if nargout > 5
    t9 = 1.0./t4;
    pzi_dot = q.*t5.*t9+r.*t2.*t9;
end
end

== matlab function modelsimulator/ROV2/ROVSubsystem/ROV ==
  data: u input; u_dot output; v input; w input; p input; q input; r input; x input; y input; z input; phi input; theta input; pzi input; tau1 input; tau2 input; tau3 input; tau4 input; tau5 input; tau6 input; v_dot output; w_dot output; p_dot output; q_dot output; r_dot output
function [u_dot,v_dot,w_dot,p_dot,q_dot,r_dot] = ROV(u,v,w,p,q,r,x,y,z,phi,theta,pzi,tau1,tau2,tau3,tau4,tau5,tau6)
%#codegen

%    This function was generated by the Symbolic Math Toolbox version 23.2.
%    07-Jun-2024 11:07:46

% u = complex(u);  % if required to enforce complex operations
% v = complex(v);  % if required to enforce complex operations
% w = complex(w);  % if required to enforce complex operations
% p = complex(p);  % if required to enforce complex operations
% q = complex(q);  % if required to enforce complex operations
% r = complex(r);  % if required to enforce complex operations
% x = complex(x);  % if required to enforce complex operations
% y = complex(y);  % if required to enforce complex operations
% z = complex(z);  % if required to enforce complex operations
% phi = complex(phi);  % if required to enforce complex operations
% theta = complex(theta);  % if required to enforce complex operations
% pzi = complex(pzi);  % if required to enforce complex operations
% tau1 = complex(tau1);  % if required to enforce complex operations
% tau2 = complex(tau2);  % if required to enforce complex operations
% tau3 = complex(tau3);  % if required to enforce complex operations
% tau4 = complex(tau4);  % if required to enforce complex operations
% tau5 = complex(tau5);  % if required to enforce complex operations
% tau6 = complex(tau6);  % if required to enforce complex operations
u_dot = tau1.*(5.0e+1./9.93e+2)-u.*(6.85e+2./9.93e+2)-q.*w.*1.620845921450151+r.*v.*1.038318227593152-u.*abs(u).*7.099697885196375;
if nargout > 1
    v_dot = tau2.*4.849425343096843e-2+p.*w.*1.561030017942874-r.*u.*9.63095873139033e-1-v.*abs(v).*1.052325299452015e+1;
end
if nargout > 2
    w_dot = tau3.*3.106554830692762e-2-w.*1.025163094128611-p.*v.*6.406026716371544e-1+q.*u.*6.169617893755825e-1-w.*abs(w).*5.902454178316247;
end
if nargout > 3
    p_dot = tau4.*2.243158366980709-cos(theta).*sin(phi).*2.973755047106326-q.*r.*5.085240017945267e-1-v.*w.*2.595109914759982e+1-p.*abs(p).*2.673844773441005;
end
if nargout > 4
    q_dot = q.*(-1.25e+2./5.7e+1)+tau5.*(6.25e+2./2.28e+2)-sin(theta).*3.634046052631579+p.*r.*3.993969298245614e-1+u.*w.*3.379934210526316e+1-q.*abs(q).*1.288377192982456;
end
if nargout > 5
    r_dot = tau6.*1.69061707523246+p.*q.*1.369399830938292e-1-u.*v.*1.286559594251902-r.*abs(r).*2.53592561284869;
end
end

== matlab function modelsimulator/Thrusters_model3/MATLAB Function9 ==
  data: u input; F output; Thruster_voltage input
function F = fcn(u,Thruster_voltage)
if Thruster_voltage == 10
    p = [-92.7173526709009	-4.21942992652299	225.484550494853	8.63193834440817	-201.940923421530	-6.79855430208119	89.8300206612197	5.42728991500474	5.00491978379944	-0.00];
elseif Thruster_voltage == 12
    p = [-102.848572308239	-7.53059973031176	248.621713648981	14.4941570056757	-222.949976245640	-9.82587357024907	101.816137648126	6.80722654001185	7.78963212289893	-0.00];
elseif Thruster_voltage == 14
    p = [-111.940783464042	-6.65861599537878	269.823430407384	13.8659958797022	-243.064927768226	-10.2880091499065	114.063389337106	8.09188399656116	10.6145211900378	-0.00];
elseif Thruster_voltage == 16
    p =  [-148.575215521583	-6.01951344606880	347.062027953365	14.7939725163702	-299.865931981745	-13.0166356354772	134.177990099770	10.1629233711657	12.7092879704266	-0.00];
elseif Thruster_voltage == 18
    p = [-162.288059231193	-9.51335388922301	365.972527557958	19.4413549873700	-302.179637889150	-11.4404685775311	136.049916333434	8.61090564659817	14.1180490642860	-0.00];
elseif Thruster_voltage == 20
    p = [-125.691529893755	-8.50647884753240	275.922008410927	13.4112646958028	-226.567986780204	-3.28875901062827	118.657519470084	6.62648580653865	14.9826070833980	0.00];
else
    p = [0];
end
F = polyval(p,u);

== matlab function modelsimulator/Subsystem2/MATLAB Function9 ==
  data: u input; F output; Thruster_voltage input
function F = fcn(u,Thruster_voltage)
if Thruster_voltage == 10
    p = [-92.7173526709009	-4.21942992652299	225.484550494853	8.63193834440817	-201.940923421530	-6.79855430208119	89.8300206612197	5.42728991500474	5.00491978379944	-0.00];
elseif Thruster_voltage == 12
    p = [-102.848572308239	-7.53059973031176	248.621713648981	14.4941570056757	-222.949976245640	-9.82587357024907	101.816137648126	6.80722654001185	7.78963212289893	-0.00];
elseif Thruster_voltage == 14
    p = [-111.940783464042	-6.65861599537878	269.823430407384	13.8659958797022	-243.064927768226	-10.2880091499065	114.063389337106	8.09188399656116	10.6145211900378	-0.00];
elseif Thruster_voltage == 16
    p =  [-148.575215521583	-6.01951344606880	347.062027953365	14.7939725163702	-299.865931981745	-13.0166356354772	134.177990099770	10.1629233711657	12.7092879704266	-0.00];
elseif Thruster_voltage == 18
    p = [-162.288059231193	-9.51335388922301	365.972527557958	19.4413549873700	-302.179637889150	-11.4404685775311	136.049916333434	8.61090564659817	14.1180490642860	-0.00];
elseif Thruster_voltage == 20
    p = [-125.691529893755	-8.50647884753240	275.922008410927	13.4112646958028	-226.567986780204	-3.28875901062827	118.657519470084	6.62648580653865	14.9826070833980	0.00];
else
    p = [0];
end
F = polyval(p,u);

== matlab function modelsimulator/Subsystem3/MATLAB Function9 ==
  data: u input; F output; Thruster_voltage input
function F = fcn(u,Thruster_voltage)
if Thruster_voltage == 10
    p = [-92.7173526709009	-4.21942992652299	225.484550494853	8.63193834440817	-201.940923421530	-6.79855430208119	89.8300206612197	5.42728991500474	5.00491978379944	-0.00];
elseif Thruster_voltage == 12
    p = [-102.848572308239	-7.53059973031176	248.621713648981	14.4941570056757	-222.949976245640	-9.82587357024907	101.816137648126	6.80722654001185	7.78963212289893	-0.00];
elseif Thruster_voltage == 14
    p = [-111.940783464042	-6.65861599537878	269.823430407384	13.8659958797022	-243.064927768226	-10.2880091499065	114.063389337106	8.09188399656116	10.6145211900378	-0.00];
elseif Thruster_voltage == 16
    p =  [-148.575215521583	-6.01951344606880	347.062027953365	14.7939725163702	-299.865931981745	-13.0166356354772	134.177990099770	10.1629233711657	12.7092879704266	-0.00];
elseif Thruster_voltage == 18
    p = [-162.288059231193	-9.51335388922301	365.972527557958	19.4413549873700	-302.179637889150	-11.4404685775311	136.049916333434	8.61090564659817	14.1180490642860	-0.00];
elseif Thruster_voltage == 20
    p = [-125.691529893755	-8.50647884753240	275.922008410927	13.4112646958028	-226.567986780204	-3.28875901062827	118.657519470084	6.62648580653865	14.9826070833980	0.00];
else
    p = [0];
end
F = polyval(p,u);

== matlab function modelsimulator/Subsystem4/MATLAB Function9 ==
  data: u input; F output; Thruster_voltage input
function F = fcn(u,Thruster_voltage)
if Thruster_voltage == 10
    p = [-92.7173526709009	-4.21942992652299	225.484550494853	8.63193834440817	-201.940923421530	-6.79855430208119	89.8300206612197	5.42728991500474	5.00491978379944	-0.00];
elseif Thruster_voltage == 12
    p = [-102.848572308239	-7.53059973031176	248.621713648981	14.4941570056757	-222.949976245640	-9.82587357024907	101.816137648126	6.80722654001185	7.78963212289893	-0.00];
elseif Thruster_voltage == 14
    p = [-111.940783464042	-6.65861599537878	269.823430407384	13.8659958797022	-243.064927768226	-10.2880091499065	114.063389337106	8.09188399656116	10.6145211900378	-0.00];
elseif Thruster_voltage == 16
    p =  [-148.575215521583	-6.01951344606880	347.062027953365	14.7939725163702	-299.865931981745	-13.0166356354772	134.177990099770	10.1629233711657	12.7092879704266	-0.00];
elseif Thruster_voltage == 18
    p = [-162.288059231193	-9.51335388922301	365.972527557958	19.4413549873700	-302.179637889150	-11.4404685775311	136.049916333434	8.61090564659817	14.1180490642860	-0.00];
elseif Thruster_voltage == 20
    p = [-125.691529893755	-8.50647884753240	275.922008410927	13.4112646958028	-226.567986780204	-3.28875901062827	118.657519470084	6.62648580653865	14.9826070833980	0.00];
else
    p = [0];
end
F = polyval(p,u);

== matlab function modelsimulator/ROV/NED/calcNED ==
  data: u input; x_dot output; v input; w input; p input; q input; r input; x input; y input; z input; phi input; theta input; pzi input; y_dot output; z_dot output; phi_dot output; theta_dot output; pzi_dot output
function [x_dot,y_dot,z_dot,phi_dot,theta_dot,pzi_dot] = calcNED(u,v,w,p,q,r,x,y,z,phi,theta,pzi)
%#codegen

%    This function was generated by the Symbolic Math Toolbox version 23.2.
%    07-Jun-2024 11:07:47

% u = complex(u);  % if required to enforce complex operations
% v = complex(v);  % if required to enforce complex operations
% w = complex(w);  % if required to enforce complex operations
% p = complex(p);  % if required to enforce complex operations
% q = complex(q);  % if required to enforce complex operations
% r = complex(r);  % if required to enforce complex operations
% x = complex(x);  % if required to enforce complex operations
% y = complex(y);  % if required to enforce complex operations
% z = complex(z);  % if required to enforce complex operations
% phi = complex(phi);  % if required to enforce complex operations
% theta = complex(theta);  % if required to enforce complex operations
% pzi = complex(pzi);  % if required to enforce complex operations
t2 = cos(phi);
t3 = cos(pzi);
t4 = cos(theta);
t5 = sin(phi);
t6 = sin(pzi);
t7 = sin(theta);
x_dot = -v.*(t2.*t6-t3.*t5.*t7)+w.*(t5.*t6+t2.*t3.*t7)+t3.*t4.*u;
if nargout > 1
    y_dot = v.*(t2.*t3+t5.*t6.*t7)-w.*(t3.*t5-t2.*t6.*t7)+t4.*t6.*u;
end
if nargout > 2
    z_dot = -t7.*u+t4.*t5.*v+t2.*t4.*w;
end
if nargout > 3
    t8 = tan(theta);
    phi_dot = p+q.*t5.*t8+r.*t2.*t8;
end
if nargout > 4
    theta_dot = q.*t2-r.*t5;
end
if nargout > 5
    t9 = 1.0./t4;
    pzi_dot = q.*t5.*t9+r.*t2.*t9;
end
end

== matlab function modelsimulator/ROV/ROVSubsystem/ROV ==
  data: u input; u_dot output; v input; w input; p input; q input; r input; x input; y input; z input; phi input; theta input; pzi input; tau1 input; tau2 input; tau3 input; tau4 input; tau5 input; tau6 input; v_dot output; w_dot output; p_dot output; q_dot output; r_dot output
function [u_dot,v_dot,w_dot,p_dot,q_dot,r_dot] = ROV(u,v,w,p,q,r,x,y,z,phi,theta,pzi,tau1,tau2,tau3,tau4,tau5,tau6)
%#codegen

%    This function was generated by the Symbolic Math Toolbox version 23.2.
%    07-Jun-2024 11:07:45

% u = complex(u);  % if required to enforce complex operations
% v = complex(v);  % if required to enforce complex operations
% w = complex(w);  % if required to enforce complex operations
% p = complex(p);  % if required to enforce complex operations
% q = complex(q);  % if required to enforce complex operations
% r = complex(r);  % if required to enforce complex operations
% x = complex(x);  % if required to enforce complex operations
% y = complex(y);  % if required to enforce complex operations
% z = complex(z);  % if required to enforce complex operations
% phi = complex(phi);  % if required to enforce complex operations
% theta = complex(theta);  % if required to enforce complex operations
% pzi = complex(pzi);  % if required to enforce complex operations
% tau1 = complex(tau1);  % if required to enforce complex operations
% tau2 = complex(tau2);  % if required to enforce complex operations
% tau3 = complex(tau3);  % if required to enforce complex operations
% tau4 = complex(tau4);  % if required to enforce complex operations
% tau5 = complex(tau5);  % if required to enforce complex operations
% tau6 = complex(tau6);  % if required to enforce complex operations
u_dot = tau1.*(5.0e+1./9.93e+2)-u.*(6.85e+2./9.93e+2)-q.*w.*1.620845921450151+r.*v.*1.038318227593152-u.*abs(u).*7.099697885196375;
if nargout > 1
    v_dot = tau2.*4.849425343096843e-2+p.*w.*1.561030017942874-r.*u.*9.63095873139033e-1-v.*abs(v).*1.052325299452015e+1;
end
if nargout > 2
    w_dot = tau3.*3.106554830692762e-2-w.*1.025163094128611-p.*v.*6.406026716371544e-1+q.*u.*6.169617893755825e-1-w.*abs(w).*5.902454178316247;
end
if nargout > 3
    p_dot = tau4.*2.243158366980709-cos(theta).*sin(phi).*2.973755047106326-q.*r.*5.085240017945267e-1-v.*w.*2.595109914759982e+1-p.*abs(p).*2.673844773441005;
end
if nargout > 4
    q_dot = q.*(-1.25e+2./5.7e+1)+tau5.*(6.25e+2./2.28e+2)-sin(theta).*3.634046052631579+p.*r.*3.993969298245614e-1+u.*w.*3.379934210526316e+1-q.*abs(q).*1.288377192982456;
end
if nargout > 5
    r_dot = tau6.*1.69061707523246+p.*q.*1.369399830938292e-1-u.*v.*1.286559594251902-r.*abs(r).*2.53592561284869;
end
end
